simulink model "non_linear_system"  (R2025b)
settings: Solver=VariableStepAuto  StartTime=0.0  StopTime=10.0  RelTol=1e-9  AbsTol=1e-9
undefined symbols (not defined in the file): b, c, g, I, l, m, M
settings Model: Creator=louisdavid  LastModifiedBy=louisdavid

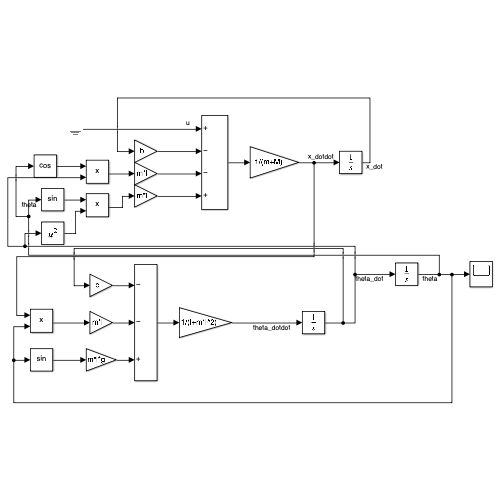
[thumbnail: Simulink's stored preview of the top-level diagram]
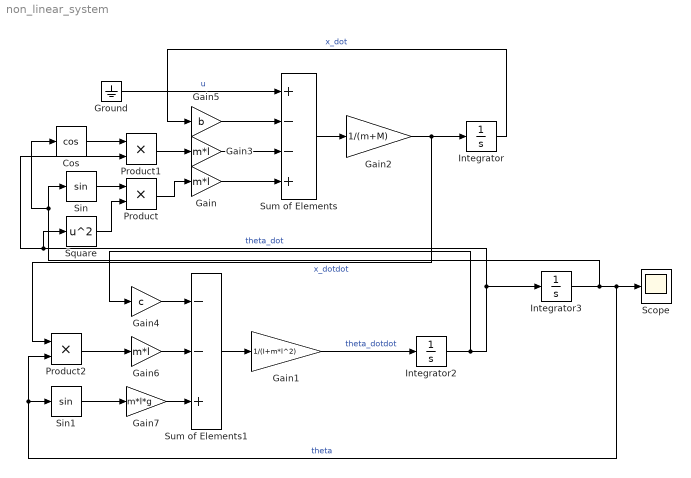
== system non_linear_system ==
  Cos : Trigonometry  Operator=cos
  Gain : Gain  Gain=m*l
  Gain1 : Gain  Gain=1/(I+m*l^2)
  Gain2 : Gain  Gain=1/(m+M)
  Gain3 : Gain  Gain=m*l
  Gain4 : Gain  Gain=c
  Gain5 : Gain  Gain=b
  Gain6 : Gain  Gain=m*l
  Gain7 : Gain  Gain=m*l*g
  Ground : Ground
  Integrator : Integrator
  Integrator2 : Integrator
  Integrator3 : Integrator  InitialCondition=15*pi/180
  Product : Product
  Product1 : Product
  Product2 : Product
  Scope : Scope
      settings: ActiveDisplayYMinimum=-6.8239018329000452  ActiveDisplayYMaximum=17.059604050291036
  Sin : Trigonometry
  Sin1 : Trigonometry
  Square : Math  Operator=square
  Sum of Elements : Sum  Inputs=+--+
  Sum of Elements1 : Sum  Inputs=--+
  wires:
  Gain2/1 -> Product2/1, Integrator/1  "x_dotdot"
  Integrator/1 -> Gain5/1  "x_dot"
  Integrator3/1 -> Cos/1, Sin/1, Product2/2, Sin1/1, Scope/1  "theta"
  Integrator2/1 -> Gain4/1, Square/1, Product1/2, Integrator3/1  "theta_dot"
  Gain1/1 -> Integrator2/1  "theta_dotdot"
  Sum of Elements/1 -> Gain2/1
  Ground/1 -> Sum of Elements/1  "u"
  Gain5/1 -> Sum of Elements/2
  Gain3/1 -> Sum of Elements/3
  Gain/1 -> Sum of Elements/4
  Product1/1 -> Gain3/1
  Cos/1 -> Product1/1
  Product/1 -> Gain/1
  Sin/1 -> Product/1
  Square/1 -> Product/2
  Sum of Elements1/1 -> Gain1/1
  Gain4/1 -> Sum of Elements1/1
  Gain6/1 -> Sum of Elements1/2
  Gain7/1 -> Sum of Elements1/3
  Sin1/1 -> Gain7/1
  Product2/1 -> Gain6/1
